simulink model "final_simulation"  (R2021b)
settings: Solver=ode8  StartTime=0.0  StopTime=T  FixedStep=0.1  RelTol=1e-3
values from neighbouring files (symbols this model uses):
  a_vec = 1./varVec    [variables.m]
  cutoff_omega = 0.1    [variables.m]
  date = date2jd([2021,2,23,0,0,0])    [variables.m]
  invJ = inv(J)    [variables.m]
  invJr = inv(Jr)    [variables.m]
  J = [Ixx 0 0; 0 Iyy 0; 0 0 Izz]    [variables.m]
  Jr = [Ir 0 0; 0 Ir 0; 0 0 Ir]    [variables.m]
  kd = 0    [variables.m]
  kdp = 0    [variables.m]
  ki = 0    [variables.m]
  kip = 1    [variables.m]
  komega = 0.01    [variables.m]
  kp = 20    [variables.m]
  kp1 = 0.2    [variables.m]
  kp2 = 2    [variables.m]
  kpp = 10    [variables.m]
  m_MT = 200    [variables.m]
  mu = astroConstants(13)    [variables.m]
  omega0 = [omegax0 omegay0 omegaz0]'    [variables.m]
  omegar0 = [omegaxr0 omegayr0 omegazr0]'    [variables.m]
  p = [0.05 0.05 0.05]'    [variables.m]
  q0 = [0 0 0 1]'    [variables.m]
  SstarsRef = [1/sqrt(3) 1 0; 1/sqrt(3) 0 1; 1/sqrt(3) 0 0]    [variables.m]
  theta0 = 2*atan(sqrt((1+en)/(1-en))*tan(E/2))    [variables.m]
undefined symbols (not defined in the file or in its folder): DiscIntNeverNeededParam, i, OM, om
libraries: matrix_library x7, my_math_ops x7, environment x5, simulink x4, vrlib x2, orbit x2, SENSORS x2, STATIC_ATT_DET x1, kinematic_transform x1
settings Model: Creator=paolo  LastModifiedBy=Davide

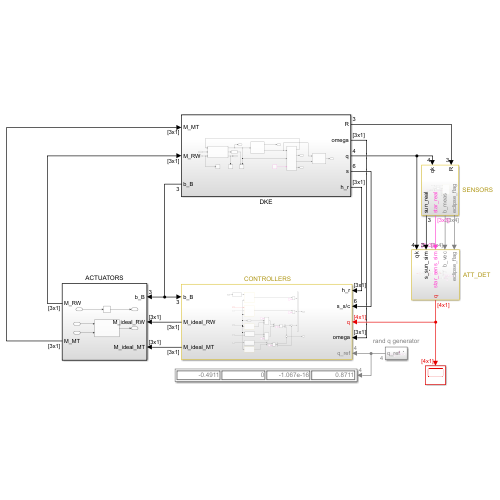
[thumbnail: Simulink's stored preview of the top-level diagram]
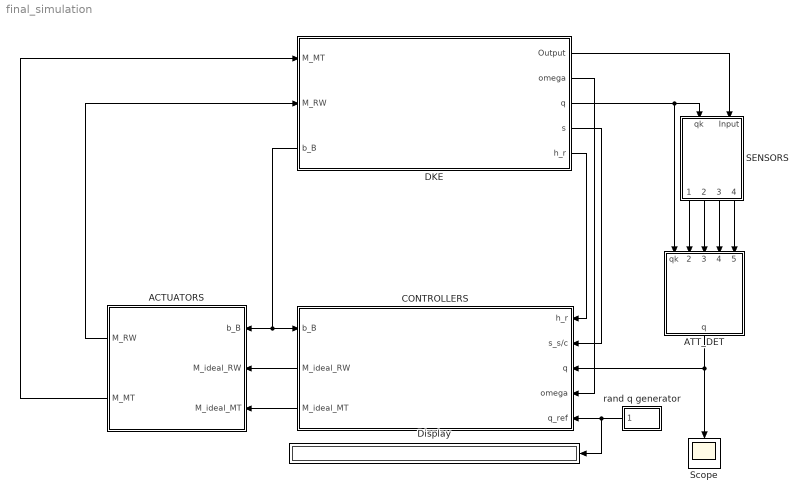
== system final_simulation ==
  " CONTROLLERS" : Subsystem
      settings: PortSchema="{\"entries\":[{\"content\":{\"sides\":[{\"content\":{\"connectorIds\":[\"In1\",\"In2\",\"In3\",\"In4\",\"In5\"]},\"type\":\"ConnectorPlacement.EquallySpacedRectSide\",\"uuid\":\"7eef0a68-69c2-4999-9870-ee920e7db8bb\"},{\"content\":{\"connectorIds\":[\"In6\",\"Out1\",\"Out2\"],\"side\":\"RIGHT\"},\"type\":\"ConnectorPlacement.EquallySpacedRectSide\",\"uuid\":\"b3de6d2c-2701-4d2f-a412-bdd263d79537\"},{\"content\":{\"connectorIds\":[],\"side\":\"TOP\"},\"type\":\"ConnectorPlacement.EquallySpacedRectSide\",\"uuid\":\"07183a01-e4e6-4ff7-8c71-3490d9a201db\"}]},\"type\":\"ConnectorPlacement.EquallySpacedConnector\",\"uuid\":\"cdaedd78-7c02-4158-8a0c-2b1dd6bc142b\"}],\"packageUris\":[\"http://schema.mathworks.com/mf0/Connector/R2020b\"],\"version\":\"1.0\"}"
  ACTUATORS : Subsystem
  ATT_DET : Subsystem
  DKE : Subsystem
      settings: PortSchema="{\"entries\":[{\"content\":{\"sides\":[{\"content\":{\"connectorIds\":[\"In1\",\"In2\",\"Out6\"]},\"type\":\"ConnectorPlacement.EquallySpacedRectSide\",\"uuid\":\"569b6a85-cacc-4d6a-9063-c3b1cb76f95a\"},{\"content\":{\"connectorIds\":[\"Out1\",\"Out2\",\"Out3\",\"Out4\",\"Out5\"],\"side\":\"RIGHT\"},\"type\":\"ConnectorPlacement.EquallySpacedRectSide\",\"uuid\":\"c98c0bd3-c24b-4331-a1c4-85d34b4b1026\"},{\"content\":{\"connectorIds\":[],\"side\":\"TOP\"},\"type\":\"ConnectorPlacement.EquallySpacedRectSide\",\"uuid\":\"0d550e56-de8b-41bd-9d95-3a45f35f27e4\"}]},\"type\":\"ConnectorPlacement.EquallySpacedConnector\",\"uuid\":\"b9a110d8-eb7f-46ee-8312-1f7318af1496\"}],\"packageUris\":[\"http://schema.mathworks.com/mf0/Connector/R2020b\"],\"version\":\"1.0\"}"
  Display : Display
  SENSORS : Subsystem
  Scope : Scope
  rand q generator : Subsystem
  wires:
  " CONTROLLERS"/2(M_ideal_MT) -> ACTUATORS/3(M_ideal_MT)
  DKE/2(omega) -> " CONTROLLERS"/4(omega)
  DKE/5(h_r) -> " CONTROLLERS"/1(h_r)
  DKE/3(q) -> ATT_DET/1(qk), SENSORS/1(qk)
  ACTUATORS/2(M_MT) -> DKE/1(M_MT)
  " CONTROLLERS"/1(M_ideal_RW) -> ACTUATORS/2(M_ideal_RW)
  DKE/6(b_B) -> ACTUATORS/1(b_B), " CONTROLLERS"/6(b_B)
  DKE/4(s) -> " CONTROLLERS"/2(s_s/c)
  ACTUATORS/1(M_RW) -> DKE/2(M_RW)
  ATT_DET/1(q) -> " CONTROLLERS"/3(q), Scope/1
  rand q generator/1(q_ref) -> " CONTROLLERS"/5(q_ref), Display/1
  SENSORS/1(sun_real) -> ATT_DET/2(s_sun_sim)
  SENSORS/2(star_real) -> ATT_DET/3(star_sens_sim)
  SENSORS/3(b_meas) -> ATT_DET/4(b_vec)
  DKE/1(Output) -> SENSORS/2(Input)
  SENSORS/4(Output) -> ATT_DET/5(Input)

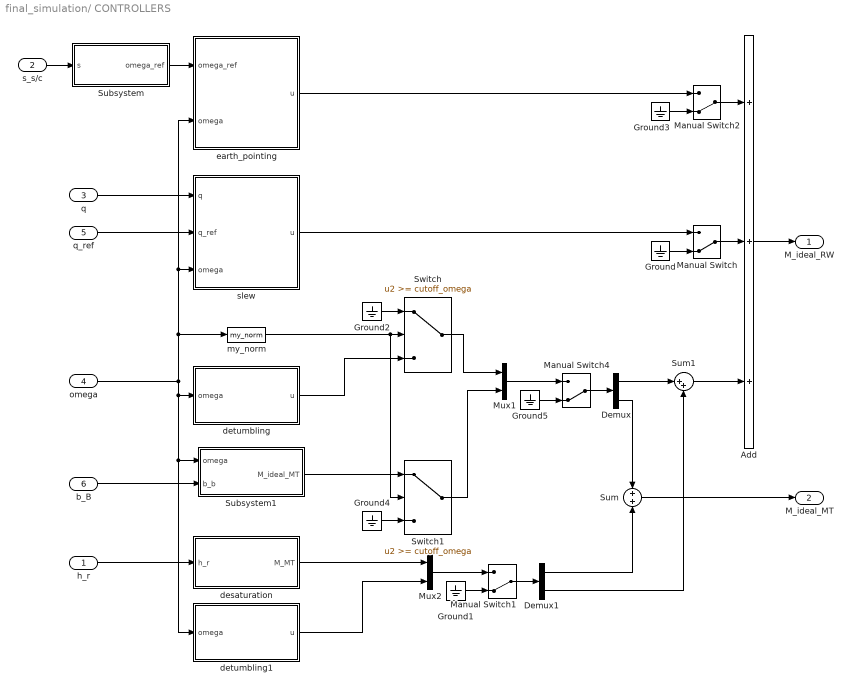
== system final_simulation/ CONTROLLERS ==
  h_r : Inport
  s_s/c : Inport  Port=2
  q : Inport  Port=3
  omega : Inport  Port=4
  q_ref : Inport  Port=5
  b_B : Inport  Port=6
  Add : Sum  Inputs=+++
  Demux : Demux  Outputs=2
  Demux1 : Demux  Outputs=2
  Ground{,1..5} (6 alike) : Ground
  Manual Switch{,1..2,4} (4 alike) : ManualSwitch  CurrentSetting=0
  Mux1 : Mux  Inputs=2
  Mux2 : Mux  Inputs=2
  Subsystem : Subsystem
  Subsystem1 : Subsystem
  Sum : Sum  Inputs=+|+
  Sum1 : Sum  Inputs=|++
  Switch : Switch  Threshold=cutoff_omega
  Switch1 : Switch  Threshold=cutoff_omega  ZeroCross=off
  desaturation : Subsystem
  detumbling : Subsystem
  detumbling1 : Subsystem
  earth_pointing : Subsystem
  my_norm : my_math_ops/my_norm  SystemSampleTime=-1  VariantActivationTime=update diagram  Latency=0  AutoFrameSizeCalculation=off
      settings: SourceProductName=My Mathematics Operations
  slew : Subsystem
  M_ideal_RW : Outport
  M_ideal_MT : Outport  Port=2
  wires:
  omega/1 -> detumbling/1(omega), detumbling1/1(omega), Subsystem1/1(omega), my_norm/1, earth_pointing/2(omega), slew/3(omega)
  Ground/1 -> Manual Switch/2
  Manual Switch/1 -> Add/2
  Add/1 -> M_ideal_RW/1
  q/1 -> slew/1(q)
  q_ref/1 -> slew/2(q_ref)
  slew/1(u) -> Manual Switch/1
  Ground3/1 -> Manual Switch2/2
  Manual Switch2/1 -> Add/1
  Subsystem/1(omega_ref) -> earth_pointing/1(omega_ref)
  earth_pointing/1(u) -> Manual Switch2/1
  s_s/c/1 -> Subsystem/1(s)
  Ground2/1 -> Switch/1
  my_norm/1 -> Switch1/2, Switch/2
  b_B/1 -> Subsystem1/2(b_b)
  Subsystem1/1(M_ideal_MT) -> Switch1/1
  Ground4/1 -> Switch1/3
  detumbling/1(u) -> Switch/3
  Switch/1 -> Mux1/1
  Switch1/1 -> Mux1/2
  Ground5/1 -> Manual Switch4/2
  Mux1/1 -> Manual Switch4/1
  Manual Switch4/1 -> Demux/1
  Demux/2 -> Sum/1
  Sum/1 -> M_ideal_MT/1
  h_r/1 -> desaturation/1(h_r)
  Mux2/1 -> Manual Switch1/1
  Manual Switch1/1 -> Demux1/1
  Ground1/1 -> Manual Switch1/2
  desaturation/1(M_MT) -> Mux2/1
  Demux1/1 -> Sum/2
  Demux/1 -> Sum1/1
  Sum1/1 -> Add/3
  detumbling1/1(u) -> Mux2/2
  Demux1/2 -> Sum1/2

== system final_simulation/ACTUATORS ==
  b_B : Inport
  M_ideal_RW : Inport  Port=2
  M_ideal_MT : Inport  Port=3
  Saturation : Saturate  UpperLimit=0.1  LowerLimit=-0.1
  Subsystem : Subsystem
  M_RW : Outport
  M_MT : Outport  Port=2
  wires:
  M_ideal_RW/1 -> Saturation/1
  Saturation/1 -> M_RW/1
  M_ideal_MT/1 -> Subsystem/1(M_ideal_MT)
  b_B/1 -> Subsystem/2(b_B)
  Subsystem/1(M_MT) -> M_MT/1

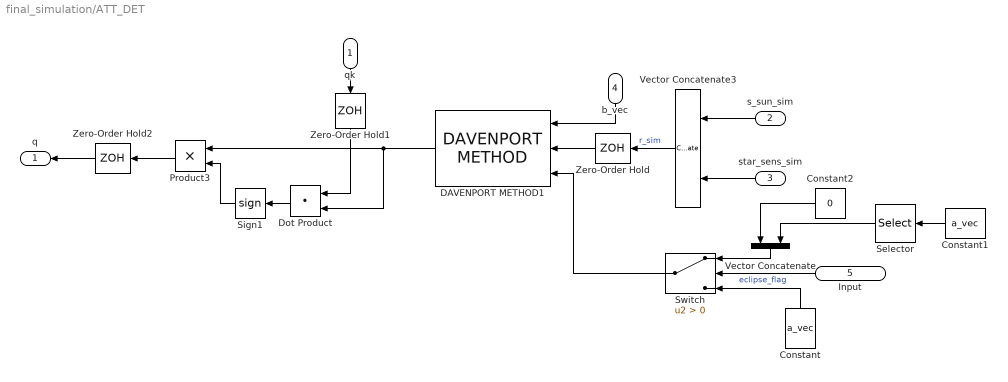
== system final_simulation/ATT_DET ==
  qk : Inport
  s_sun_sim : Inport  Port=2
  star_sens_sim : Inport  Port=3
  b_vec : Inport  Port=4
  Input : Inport  Port=5
  Constant : Constant  Value=a_vec
  Constant1 : Constant  Value=a_vec
  Constant2 : Constant  Value=0
  DAVENPORT METHOD1 : STATIC_ATT_DET/DAVENPORT METHOD  SystemSampleTime=-1  VariantActivationTime=update diagram  Latency=0  AutoFrameSizeCalculation=off
      settings: SourceProductName=Attitude Determination (static)
  Dot Product : DotProduct  InputSameDT=on  OutDataTypeStr=Inherit: Inherit via internal rule
  Product3 : Product
  Selector : Selector  InputPortWidth=4  IndexOptions=Index vector (dialog)  Indices=[2 3 4]  OutputSizes=1
  Sign1 : Signum
  Switch : Switch  Criteria=u2 > Threshold
  Vector Concatenate : Concatenate
  Vector Concatenate3 : Concatenate  Mode=Multidimensional array  ConcatenateDimension=2
  Zero-Order Hold : ZeroOrderHold  SampleTime=0.1
  Zero-Order Hold1 : ZeroOrderHold  SampleTime=0.1
  Zero-Order Hold2 : ZeroOrderHold  SampleTime=0.1
  q : Outport
  wires:
  star_sens_sim/1 -> Vector Concatenate3/2
  DAVENPORT METHOD1/1 -> Dot Product/2, Product3/1
  Sign1/1 -> Product3/2
  qk/1 -> Zero-Order Hold1/1
  Vector Concatenate3/1 -> Zero-Order Hold/1  "r_sim"
  Dot Product/1 -> Sign1/1
  s_sun_sim/1 -> Vector Concatenate3/1
  b_vec/1 -> DAVENPORT METHOD1/1
  Zero-Order Hold/1 -> DAVENPORT METHOD1/2
  Zero-Order Hold1/1 -> Dot Product/1
  Input/1 -> Switch/2  "eclipse_flag"
  Switch/1 -> DAVENPORT METHOD1/3
  Constant/1 -> Switch/3
  Constant1/1 -> Selector/1
  Selector/1 -> Vector Concatenate/2
  Constant2/1 -> Vector Concatenate/1
  Vector Concatenate/1 -> Switch/1
  Product3/1 -> Zero-Order Hold2/1
  Zero-Order Hold2/1 -> q/1

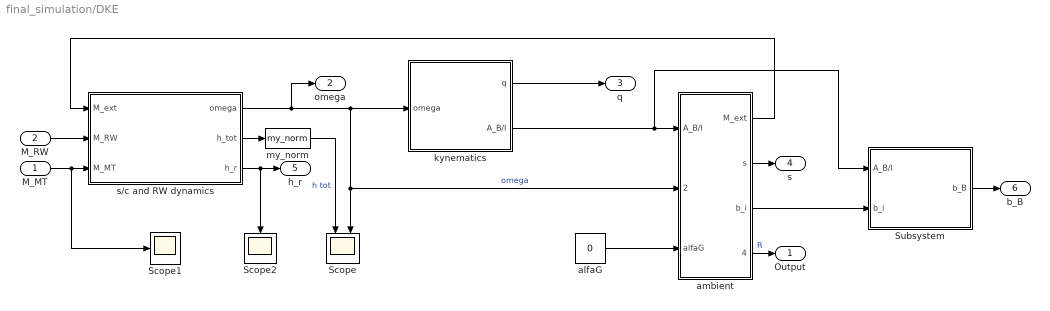
== system final_simulation/DKE ==
  M_MT : Inport
  M_RW : Inport  Port=2
  Scope : Scope  NumInputPorts=2
  Scope1 : Scope
  Scope2 : Scope
  Subsystem : Subsystem
  alfaG : Constant  Value=0
  ambient : Subsystem
  kynematics : Subsystem
  my_norm : my_math_ops/my_norm  SystemSampleTime=-1  VariantActivationTime=update diagram  Latency=0  AutoFrameSizeCalculation=off
      settings: SourceProductName=My Mathematics Operations
  s/c and RW dynamics : Subsystem
  Output : Outport
  omega : Outport  Port=2
  q : Outport  Port=3
  s : Outport  Port=4
  h_r : Outport  Port=5
  b_B : Outport  Port=6
  wires:
  s/c and RW dynamics/1(omega) -> Scope/2, ambient/2(omega), kynematics/1(omega), omega/1  "omega"
  kynematics/2(A_B/I) -> ambient/1(A_B/I), Subsystem/1(A_B/I)
  s/c and RW dynamics/2(h_tot) -> my_norm/1
  kynematics/1(q) -> q/1
  M_RW/1 -> s/c and RW dynamics/2(M_RW)
  ambient/1(M_ext) -> s/c and RW dynamics/1(M_ext)
  my_norm/1 -> Scope/1  "h tot"
  ambient/2(s) -> s/1
  alfaG/1 -> ambient/3(alfaG)
  ambient/3(b_i) -> Subsystem/2(b_i)
  M_MT/1 -> Scope1/1, s/c and RW dynamics/3(M_MT)
  Subsystem/1(b_B) -> b_B/1
  s/c and RW dynamics/3(h_r) -> Scope2/1, h_r/1
  ambient/4(Output) -> Output/1  "R"

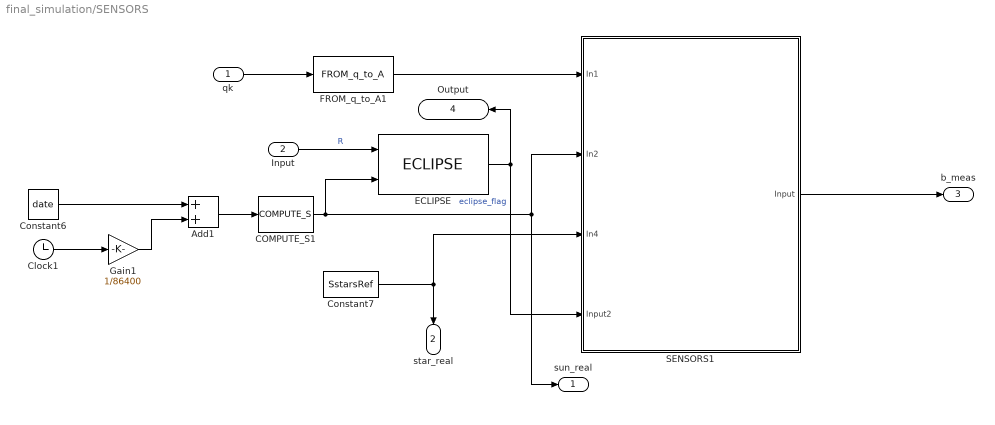
== system final_simulation/SENSORS ==
  qk : Inport
  Input : Inport  Port=2
  Add1 : Sum
  COMPUTE_S1 : environment/COMPUTE_S  SystemSampleTime=-1  VariantActivationTime=update diagram  Latency=0  AutoFrameSizeCalculation=off
      settings: SourceProductName=Environment
  Clock1 : Clock
  Constant6 : Constant  Value=date
  Constant7 : Constant  Value=SstarsRef
  ECLIPSE : environment/ECLIPSE  SystemSampleTime=-1  VariantActivationTime=update diagram  Latency=0  AutoFrameSizeCalculation=off
      settings: SourceProductName=Environment
  FROM_q_to_A1 : kinematic_transform/FROM_q_to_A  SystemSampleTime=-1  VariantActivationTime=update diagram  Latency=0  AutoFrameSizeCalculation=off
      settings: SourceProductName=Kinematic Transformation
  Gain1 : Gain  Gain=1/86400
  SENSORS1 : Subsystem
  sun_real : Outport
  star_real : Outport  Port=2
  b_meas : Outport  Port=3
  Output : Outport  Port=4
  wires:
  Gain1/1 -> Add1/2
  Constant7/1 -> star_real/1, SENSORS1/3(In4)
  Constant6/1 -> Add1/1
  FROM_q_to_A1/1 -> SENSORS1/1(In1)
  Add1/1 -> COMPUTE_S1/1
  Clock1/1 -> Gain1/1
  SENSORS1/1(Input) -> b_meas/1
  COMPUTE_S1/1 -> ECLIPSE/2, sun_real/1, SENSORS1/2(In2)
  qk/1 -> FROM_q_to_A1/1
  Input/1 -> ECLIPSE/1  "R"
  ECLIPSE/1 -> SENSORS1/4(Input2), Output/1  "eclipse_flag"

== system final_simulation/rand q generator ==
  Compare To Zero : simulink/Logic and Bit Operations/Compare To Zero  relop=>=  OutDataTypeStr=boolean
  Constant4 : Constant  Value=[rand(4,1)]
  Constant5 : Constant  Value=q0
  Constant8 : Constant  Value=randi([-1 1],4,1)
  Constant9 : Constant
  Gain2 : Gain  Gain=2
  Manual Switch : ManualSwitch
  Normalize Vector1 : vrlib/Utilities/Normalize Vector  maxzero=0
  Product2 : Product
  Subtract : Sum  Inputs=+-
  q_ref : Outport
  wires:
  Constant4/1 -> Normalize Vector1/1
  Normalize Vector1/1 -> Product2/1
  Constant8/1 -> Compare To Zero/1
  Constant9/1 -> Subtract/2
  Subtract/1 -> Product2/2
  Compare To Zero/1 -> Gain2/1
  Gain2/1 -> Subtract/1
  Manual Switch/1 -> q_ref/1
  Constant5/1 -> Manual Switch/2
  Product2/1 -> Manual Switch/1

== system final_simulation/ CONTROLLERS/Subsystem ==
  s : Inport
  Cross Product : matrix_library/Cross Product
      settings: SourceProductBaseCode=SL
  Demux : Demux  Outputs=2
  Divide : Product  Inputs=/*
  Ground : Ground
  Ground1 : Ground
  Mux : Mux  Inputs=3
  Scope : Scope
  Square : Math  Operator=square  SaturateOnIntegerOverflow=on
  my_norm : my_math_ops/my_norm  SystemSampleTime=-1  VariantActivationTime=update diagram  Latency=0  AutoFrameSizeCalculation=off
      settings: SourceProductName=My Mathematics Operations
  my_norm1 : my_math_ops/my_norm  SystemSampleTime=-1  VariantActivationTime=update diagram  Latency=0  AutoFrameSizeCalculation=off
      settings: SourceProductName=My Mathematics Operations
  omega_ref : Outport
  wires:
  s/1 -> Demux/1
  Demux/1 -> my_norm/1, Cross Product/1  "R"
  Demux/2 -> Cross Product/2  "V"
  Cross Product/1 -> my_norm1/1
  my_norm/1 -> Scope/1, Square/1
  Square/1 -> Divide/1
  my_norm1/1 -> Divide/2
  Mux/1 -> omega_ref/1
  Divide/1 -> Mux/3
  Ground/1 -> Mux/1
  Ground1/1 -> Mux/2

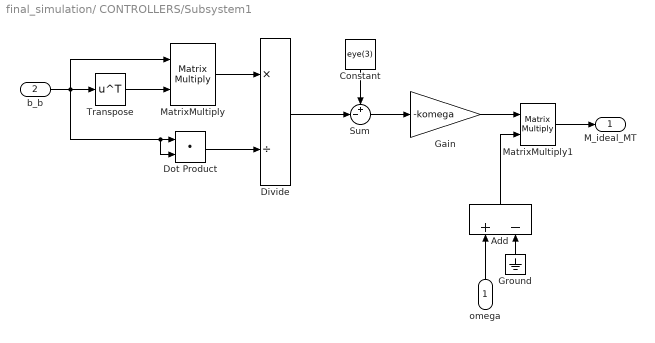
== system final_simulation/ CONTROLLERS/Subsystem1 ==
  omega : Inport
  b_b : Inport  Port=2
  Add : Sum  Inputs=+-
  Constant : Constant  Value=eye(3)
  Divide : Product  Inputs=*/
  Dot Product : DotProduct  InputSameDT=on  OutDataTypeStr=Inherit: Inherit via internal rule
  Gain : Gain  Gain=-komega
  Ground : Ground
  MatrixMultiply : Product  Multiplication=Matrix(*)
  MatrixMultiply1 : Product  Multiplication=Matrix(*)
  Sum : Sum  Inputs=+-|
  Transpose : Math  Operator=transpose  SaturateOnIntegerOverflow=on
  M_ideal_MT : Outport
  wires:
  Ground/1 -> Add/2
  omega/1 -> Add/1
  b_b/1 -> Dot Product/2, Dot Product/1, MatrixMultiply/1, Transpose/1
  Transpose/1 -> MatrixMultiply/2
  MatrixMultiply/1 -> Divide/1
  Dot Product/1 -> Divide/2
  Constant/1 -> Sum/1
  Divide/1 -> Sum/2
  Sum/1 -> Gain/1
  MatrixMultiply1/1 -> M_ideal_MT/1
  Gain/1 -> MatrixMultiply1/1
  Add/1 -> MatrixMultiply1/2

== system final_simulation/ CONTROLLERS/desaturation ==
  h_r : Inport
  Abs : Abs
  Constant : Constant
  Divide : Product  Inputs=*/
  Gain : Gain  Gain=-1/10
  MatrixMultiply : Product
  M_MT : Outport
  wires:
  Constant/1 -> Divide/1
  Divide/1 -> Abs/1
  Abs/1 -> MatrixMultiply/2
  MatrixMultiply/1 -> Gain/1
  h_r/1 -> MatrixMultiply/1, Divide/2
  Gain/1 -> M_MT/1

== system final_simulation/ CONTROLLERS/detumbling ==
  omega : Inport
  Add : Sum  Inputs=+-
  Discrete Derivative : simulink/Discrete/Discrete Derivative  gainval=1.0  ICPrevScaledInput=0.0  OutMin=[]  OutMax=[]  OutDataType=fixdt(1, 16)  OutScaling=2^-10  DoSatur=off
  Discrete-Time Integrator : DiscreteIntegrator  SampleTime=-1  ICPrevOutput=DiscIntNeverNeededParam  ICPrevScaledInput=DiscIntNeverNeededParam
  Gain : Gain  Gain=kp
  Gain1 : Gain  Gain=ki
  Gain2 : Gain  Gain=kd
  Ground : Ground
  Sum2 : Sum  Inputs=---
  u : Outport
  wires:
  Add/1 -> Gain/1, Discrete Derivative/1, Discrete-Time Integrator/1
  Ground/1 -> Add/2
  omega/1 -> Add/1
  Gain/1 -> Sum2/2
  Gain2/1 -> Sum2/3
  Gain1/1 -> Sum2/1
  Discrete-Time Integrator/1 -> Gain1/1
  Discrete Derivative/1 -> Gain2/1
  Sum2/1 -> u/1

== system final_simulation/ CONTROLLERS/detumbling1 ==
  omega : Inport
  Add : Sum  Inputs=+-
  Discrete Derivative : simulink/Discrete/Discrete Derivative  gainval=1.0  ICPrevScaledInput=0.0  OutMin=[]  OutMax=[]  OutDataType=fixdt(1, 16)  OutScaling=2^-10  DoSatur=off
  Discrete-Time Integrator : DiscreteIntegrator  SampleTime=-1  ICPrevOutput=DiscIntNeverNeededParam  ICPrevScaledInput=DiscIntNeverNeededParam
  Gain : Gain  Gain=kp
  Gain1 : Gain  Gain=ki
  Gain2 : Gain  Gain=kd
  Ground : Ground
  Sum2 : Sum  Inputs=---
  u : Outport
  wires:
  Add/1 -> Gain/1, Discrete Derivative/1, Discrete-Time Integrator/1
  Ground/1 -> Add/2
  omega/1 -> Add/1
  Gain/1 -> Sum2/2
  Gain2/1 -> Sum2/3
  Gain1/1 -> Sum2/1
  Discrete-Time Integrator/1 -> Gain1/1
  Discrete Derivative/1 -> Gain2/1
  Sum2/1 -> u/1

== system final_simulation/ CONTROLLERS/earth_pointing ==
  omega_ref : Inport
  omega : Inport  Port=2
  Add : Sum  Inputs=+-
  Discrete Derivative : simulink/Discrete/Discrete Derivative  gainval=1.0  ICPrevScaledInput=0.0  OutMin=[]  OutMax=[]  OutDataType=fixdt(1, 16)  OutScaling=2^-10  DoSatur=off
  Discrete-Time Integrator : DiscreteIntegrator  SampleTime=-1  ICPrevOutput=DiscIntNeverNeededParam  ICPrevScaledInput=DiscIntNeverNeededParam
  Gain : Gain  Gain=kpp
  Gain1 : Gain  Gain=kip
  Gain2 : Gain  Gain=kdp
  Sum2 : Sum  Inputs=---
  u : Outport
  wires:
  Add/1 -> Gain/1, Discrete Derivative/1, Discrete-Time Integrator/1
  Gain/1 -> Sum2/2
  Sum2/1 -> u/1
  omega/1 -> Add/1
  Discrete-Time Integrator/1 -> Gain1/1
  Gain1/1 -> Sum2/1
  omega_ref/1 -> Add/2
  Gain2/1 -> Sum2/3
  Discrete Derivative/1 -> Gain2/1

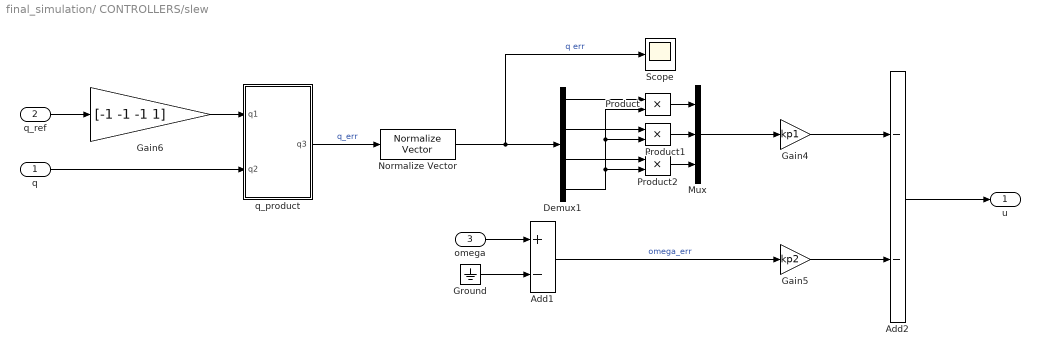
== system final_simulation/ CONTROLLERS/slew ==
  q : Inport
  q_ref : Inport  Port=2
  omega : Inport  Port=3
  Add1 : Sum  Inputs=+-
  Add2 : Sum  Inputs=--
  Demux1 : Demux
  Gain4 : Gain  Gain=kp1
  Gain5 : Gain  Gain=kp2
  Gain6 : Gain  Gain=[-1 -1 -1 1]
  Ground : Ground
  Mux : Mux  Inputs=3
  Normalize Vector : vrlib/Utilities/Normalize Vector  maxzero=0
  Product : Product
  Product1 : Product
  Product2 : Product
  Scope : Scope
  q_product : Subsystem
  u : Outport
  wires:
  omega/1 -> Add1/1
  Ground/1 -> Add1/2
  Add1/1 -> Gain5/1  "omega_err"
  Gain5/1 -> Add2/2
  Add2/1 -> u/1
  Gain4/1 -> Add2/1
  Normalize Vector/1 -> Scope/1, Demux1/1  "q err"
  Demux1/4 -> Product/2, Product1/2, Product2/2
  Mux/1 -> Gain4/1
  q_ref/1 -> Gain6/1
  Gain6/1 -> q_product/1(q1)
  q/1 -> q_product/2(q2)
  q_product/1(q3) -> Normalize Vector/1  "q_err"
  Product/1 -> Mux/1
  Product1/1 -> Mux/2
  Product2/1 -> Mux/3
  Demux1/3 -> Product2/1
  Demux1/2 -> Product1/1
  Demux1/1 -> Product/1

== system final_simulation/ACTUATORS/Subsystem ==
  M_ideal_MT : Inport
  b_B : Inport  Port=2
  Cross Product : matrix_library/Cross Product
      settings: SourceProductBaseCode=SL
  Cross Product1 : matrix_library/Cross Product
      settings: SourceProductBaseCode=SL
  Divide : Product  Inputs=*/
  Dot Product : DotProduct  InputSameDT=on  OutDataTypeStr=Inherit: Inherit via internal rule
  Saturation : Saturate  UpperLimit=m_MT  LowerLimit=-m_MT
  Scope : Scope
  Scope1 : Scope  NumInputPorts=2
  M_MT : Outport
  wires:
  b_B/1 -> Cross Product/1, Cross Product1/2, Dot Product/2, Dot Product/1  "b_B"
  M_ideal_MT/1 -> Scope1/2, Cross Product/2
  Cross Product/1 -> Divide/1
  Dot Product/1 -> Divide/2
  Cross Product1/1 -> Scope1/1, M_MT/1
  Divide/1 -> Saturation/1
  Saturation/1 -> Scope/1, Cross Product1/1  "d_B"

== system final_simulation/DKE/Subsystem ==
  A_B/I : Inport
  b_i : Inport  Port=2
  MatrixMultiply : Product  Multiplication=Matrix(*)
  b_B : Outport
  wires:
  A_B/I/1 -> MatrixMultiply/1
  b_i/1 -> MatrixMultiply/2
  MatrixMultiply/1 -> b_B/1  "b_B"

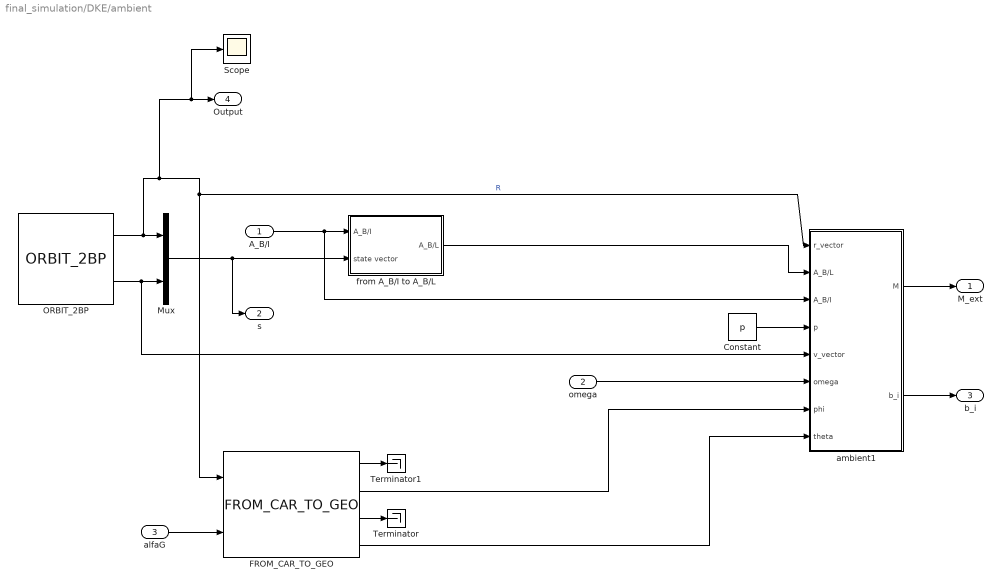
== system final_simulation/DKE/ambient ==
  A_B/I : Inport
  omega : Inport  Port=2
  alfaG : Inport  Port=3
  Constant : Constant  Value=p
  FROM_CAR_TO_GEO : orbit/FROM_CAR_TO_GEO  SystemSampleTime=-1  VariantActivationTime=update diagram  Latency=0  AutoFrameSizeCalculation=off
      settings: SourceProductName=Orbit
  Mux : Mux  Inputs=2
  ORBIT_2BP : orbit/ORBIT_2BP  SystemSampleTime=-1  VariantActivationTime=update diagram  Latency=0  AutoFrameSizeCalculation=off
      settings: SourceProductName=Orbit
  Scope : Scope
  Terminator : Terminator
  Terminator1 : Terminator
  ambient1 : Subsystem
  from A_B/I to A_B/L : Subsystem
  M_ext : Outport
  s : Outport  Port=2
  b_i : Outport  Port=3
  Output : Outport  Port=4
  wires:
  ORBIT_2BP/1 -> Scope/1, Output/1, ambient1/1(r_vector), FROM_CAR_TO_GEO/1, Mux/1  "R"
  ORBIT_2BP/2 -> ambient1/5(v_vector), Mux/2
  Mux/1 -> s/1, from A_B/I to A_B/L/2(state vector)
  A_B/I/1 -> ambient1/3(A_B/I), from A_B/I to A_B/L/1(A_B/I)
  alfaG/1 -> FROM_CAR_TO_GEO/2
  FROM_CAR_TO_GEO/3 -> Terminator/1
  FROM_CAR_TO_GEO/1 -> Terminator1/1
  ambient1/1(M) -> M_ext/1
  from A_B/I to A_B/L/1(A_B/L) -> ambient1/2(A_B/L)
  FROM_CAR_TO_GEO/2 -> ambient1/7(phi)
  FROM_CAR_TO_GEO/4 -> ambient1/8(theta)
  omega/1 -> ambient1/6(omega)
  Constant/1 -> ambient1/4(p)
  ambient1/2(b_i) -> b_i/1

== system final_simulation/DKE/kynematics ==
  omega : Inport
  kynematics q : Subsystem
  q to A_B/I : Subsystem
  q : Outport
  A_B/I : Outport  Port=2
  wires:
  omega/1 -> kynematics q/1(omega)
  kynematics q/1(q) -> q to A_B/I/1(q), q/1
  q to A_B/I/1(Aq) -> A_B/I/1

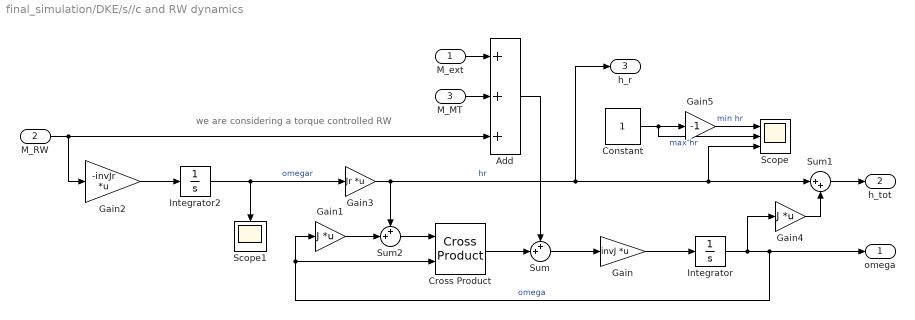
== system final_simulation/DKE/s//c and RW dynamics ==
  note: we are considering a torque controlled RW
  M_ext : Inport
  M_RW : Inport  Port=2
  M_MT : Inport  Port=3
  Add : Sum  Inputs=+++
  Constant : Constant
  Cross Product : matrix_library/Cross Product
      settings: SourceProductBaseCode=SL
  Gain : Gain  Gain=invJ  Multiplication=Matrix(K*u)
  Gain1 : Gain  Gain=J  Multiplication=Matrix(K*u)
  Gain2 : Gain  Gain=-invJr  Multiplication=Matrix(K*u)
  Gain3 : Gain  Gain=Jr  Multiplication=Matrix(K*u)
  Gain4 : Gain  Gain=J  Multiplication=Matrix(K*u)
  Gain5 : Gain  Gain=-1
  Integrator : Integrator  InitialCondition=omega0
  Integrator2 : Integrator  InitialCondition=omegar0
  Scope : Scope  NumInputPorts=3
  Scope1 : Scope
  Sum : Sum  Inputs=++|
  Sum1 : Sum  Inputs=|++
  Sum2 : Sum  Inputs=++|
  omega : Outport
  h_tot : Outport  Port=2
  h_r : Outport  Port=3
  wires:
  Integrator/1 -> omega/1, Gain1/1, Cross Product/2, Gain4/1  "omega"
  Cross Product/1 -> Sum/2
  Sum/1 -> Gain/1
  Gain/1 -> Integrator/1
  Sum2/1 -> Cross Product/1
  Gain1/1 -> Sum2/2
  M_RW/1 -> Add/3, Gain2/1
  Gain2/1 -> Integrator2/1
  Gain3/1 -> Sum2/1, Scope/3, Sum1/1, h_r/1  "hr"
  Integrator2/1 -> Gain3/1, Scope1/1  "omegar"
  Gain4/1 -> Sum1/2
  Sum1/1 -> h_tot/1
  Add/1 -> Sum/1
  Constant/1 -> Gain5/1, Scope/2  "max hr"
  M_ext/1 -> Add/1
  Gain5/1 -> Scope/1  "min hr"
  M_MT/1 -> Add/2

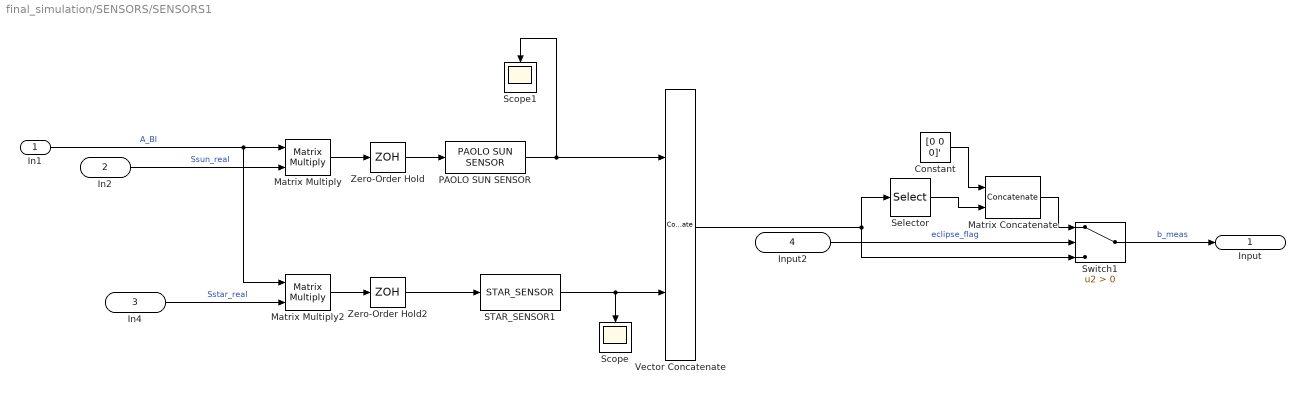
== system final_simulation/SENSORS/SENSORS1 ==
  In1 : Inport
  In2 : Inport  Port=2
  In4 : Inport  Port=3
  Input2 : Inport  Port=4
  Constant : Constant  Value=[0 0 0]'
  Matrix Concatenate : Concatenate  Mode=Multidimensional array  ConcatenateDimension=2
  Matrix Multiply : Product  Multiplication=Matrix(*)
  Matrix Multiply2 : Product  Multiplication=Matrix(*)
  PAOLO SUN SENSOR : SENSORS/PAOLO SUN SENSOR  SystemSampleTime=-1  VariantActivationTime=update diagram  Latency=0  AutoFrameSizeCalculation=off
      settings: SourceProductName=Sensors
  STAR_SENSOR1 : SENSORS/STAR_SENSOR  SystemSampleTime=-1  VariantActivationTime=update diagram  Latency=0  AutoFrameSizeCalculation=off
      settings: SourceProductName=Sensors
  Scope : Scope
  Scope1 : Scope
  Selector : Selector  NumberOfDimensions=2  InputPortWidth=3  IndexOptions=Index vector (dialog),Index vector (dialog)  Indices=[1 2 3],[2 3 4]  OutputSizes=1,1
  Switch1 : Switch  Criteria=u2 > Threshold
  Vector Concatenate : Concatenate  Mode=Multidimensional array  ConcatenateDimension=2
  Zero-Order Hold : ZeroOrderHold  SampleTime=0.1
  Zero-Order Hold2 : ZeroOrderHold  SampleTime=0.2
  Input : Outport
  wires:
  Zero-Order Hold2/1 -> STAR_SENSOR1/1
  STAR_SENSOR1/1 -> Vector Concatenate/2, Scope/1
  In1/1 -> Matrix Multiply2/1, Matrix Multiply/1  "A_BI"
  In4/1 -> Matrix Multiply2/2  "Sstar_real"
  Matrix Multiply2/1 -> Zero-Order Hold2/1
  In2/1 -> Matrix Multiply/2  "Ssun_real"
  Matrix Multiply/1 -> Zero-Order Hold/1
  Vector Concatenate/1 -> Switch1/3, Selector/1
  Zero-Order Hold/1 -> PAOLO SUN SENSOR/1
  PAOLO SUN SENSOR/1 -> Vector Concatenate/1, Scope1/1
  Input2/1 -> Switch1/2  "eclipse_flag"
  Switch1/1 -> Input/1  "b_meas"
  Selector/1 -> Matrix Concatenate/2
  Constant/1 -> Matrix Concatenate/1
  Matrix Concatenate/1 -> Switch1/1

== system final_simulation/ CONTROLLERS/slew/q_product ==
  q1 : Inport
  q2 : Inport  Port=2
  Add : Sum  Inputs=3
  Add1 : Sum  Inputs=+-
  Cross Product : matrix_library/Cross Product
      settings: SourceProductBaseCode=SL
  Dot Product : DotProduct  InputSameDT=on  OutDataTypeStr=Inherit: Inherit via internal rule
  Product : Product
  Product1 : Product
  Product2 : Product
  Subsystem : Subsystem
  Subsystem1 : Subsystem
  Vector Concatenate : Concatenate
  q3 : Outport
  wires:
  Product/1 -> Add/2
  Subsystem1/2(n_ref) -> Product1/1, Product2/2
  Subsystem/1(g) -> Dot Product/1, Product1/2, Cross Product/1
  Cross Product/1 -> Add/1
  q1/1 -> Subsystem/1(q)
  Subsystem1/1(g_ref) -> Dot Product/2, Product/2, Cross Product/2
  Add/1 -> Vector Concatenate/1
  Product1/1 -> Add/3
  Dot Product/1 -> Add1/2
  Subsystem/2(n) -> Product2/1, Product/1
  Product2/1 -> Add1/1
  Add1/1 -> Vector Concatenate/2
  q2/1 -> Subsystem1/1(q_ref)
  Vector Concatenate/1 -> q3/1

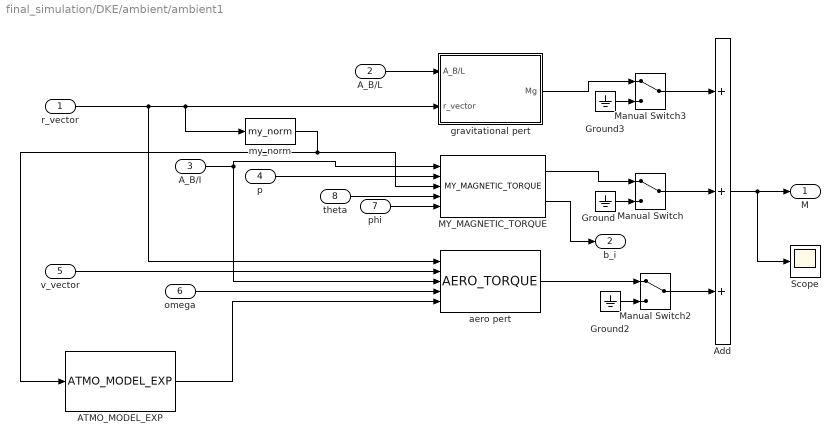
== system final_simulation/DKE/ambient/ambient1 ==
  r_vector : Inport
  A_B/L : Inport  Port=2
  A_B/I : Inport  Port=3
  p : Inport  Port=4
  v_vector : Inport  Port=5
  omega : Inport  Port=6
  phi : Inport  Port=7
  theta : Inport  Port=8
  ATMO_MODEL_EXP : environment/ATMO_MODEL_EXP  SystemSampleTime=-1  VariantActivationTime=update diagram  Latency=0  AutoFrameSizeCalculation=off
      settings: SourceProductName=Environment
  Add : Sum  Inputs=+++
  Ground : Ground
  Ground2 : Ground
  Ground3 : Ground
  MY_MAGNETIC_TORQUE : environment/MY_MAGNETIC_TORQUE  SystemSampleTime=-1  VariantActivationTime=update diagram  Latency=0  AutoFrameSizeCalculation=off
      settings: SourceProductName=Environment
  Manual Switch : ManualSwitch
  Manual Switch2 : ManualSwitch
  Manual Switch3 : ManualSwitch
  Scope : Scope
  aero pert : environment/AERO_TORQUE  SystemSampleTime=-1  VariantActivationTime=update diagram  Latency=0  AutoFrameSizeCalculation=off
      settings: SourceProductName=Environment
  gravitational pert : Subsystem
  my_norm : my_math_ops/my_norm  SystemSampleTime=-1  VariantActivationTime=update diagram  Latency=0  AutoFrameSizeCalculation=off
      settings: SourceProductName=My Mathematics Operations
  M : Outport
  b_i : Outport  Port=2
  wires:
  p/1 -> MY_MAGNETIC_TORQUE/2
  theta/1 -> MY_MAGNETIC_TORQUE/4
  ATMO_MODEL_EXP/1 -> aero pert/5
  MY_MAGNETIC_TORQUE/1 -> Manual Switch/1
  omega/1 -> aero pert/4
  phi/1 -> MY_MAGNETIC_TORQUE/5
  aero pert/1 -> Manual Switch2/1
  gravitational pert/1(Mg) -> Manual Switch3/1
  A_B/I/1 -> MY_MAGNETIC_TORQUE/1, aero pert/3
  Ground2/1 -> Manual Switch2/2
  Manual Switch/1 -> Add/2
  v_vector/1 -> aero pert/2
  Ground3/1 -> Manual Switch3/2
  Add/1 -> Scope/1, M/1
  my_norm/1 -> MY_MAGNETIC_TORQUE/3, ATMO_MODEL_EXP/1
  r_vector/1 -> aero pert/1, my_norm/1, gravitational pert/2(r_vector)
  Ground/1 -> Manual Switch/2
  Manual Switch2/1 -> Add/3
  A_B/L/1 -> gravitational pert/1(A_B/L)
  Manual Switch3/1 -> Add/1
  MY_MAGNETIC_TORQUE/2 -> b_i/1

== system final_simulation/DKE/ambient/from A_B//I to A_B//L ==
  A_B/I : Inport
  state vector : Inport  Port=2
  A_I_LVLH1 : Subsystem
  Demux : Demux  Outputs=2
  MatrixMultiply : Product  Multiplication=Matrix(*)
  Subsystem : Subsystem
  Terminator : Terminator
  A_B/L : Outport
  wires:
  MatrixMultiply/1 -> A_B/L/1
  A_B/I/1 -> MatrixMultiply/1
  A_I_LVLH1/1(Out1) -> MatrixMultiply/2  "A_I/L"
  Subsystem/2(Out2) -> Terminator/1  "omega_L"
  Subsystem/1(Out1) -> A_I_LVLH1/1(Input)
  Demux/1 -> Subsystem/1(a)
  Demux/2 -> Subsystem/2(b)
  state vector/1 -> Demux/1

== system final_simulation/DKE/kynematics/kynematics q ==
  omega : Inport
  Add : Sum  Inputs=+++
  Demux : Demux  Outputs=3
  Gain : Gain  Gain=[0 0 0 1; 0 0 1 0; 0 -1 0 0; -1 0 0 0]
  Gain1 : Gain  Gain=[0 0 -1 0; 0 0 0 1; 1 0 0 0; 0 -1 0 0]
  Gain2 : Gain  Gain=[0 1 0 0; -1 0 0 0; 0 0 0 1; 0 0 -1 0]
  Gain3 : Gain  Gain=1/2
  Integrator : Integrator  InitialCondition=q0
  Product : Product  Multiplication=Matrix(*)
  normalization : Subsystem
  q : Outport
  wires:
  Product/1 -> Integrator/1  "dq"
  Gain/1 -> Add/1
  Gain3/1 -> Product/1
  Add/1 -> Gain3/1
  Gain2/1 -> Add/3
  Gain1/1 -> Add/2
  Demux/3 -> Gain2/1
  Demux/1 -> Gain/1
  Demux/2 -> Gain1/1
  omega/1 -> Demux/1
  Integrator/1 -> normalization/1(q0)
  normalization/1(q) -> Product/2, q/1

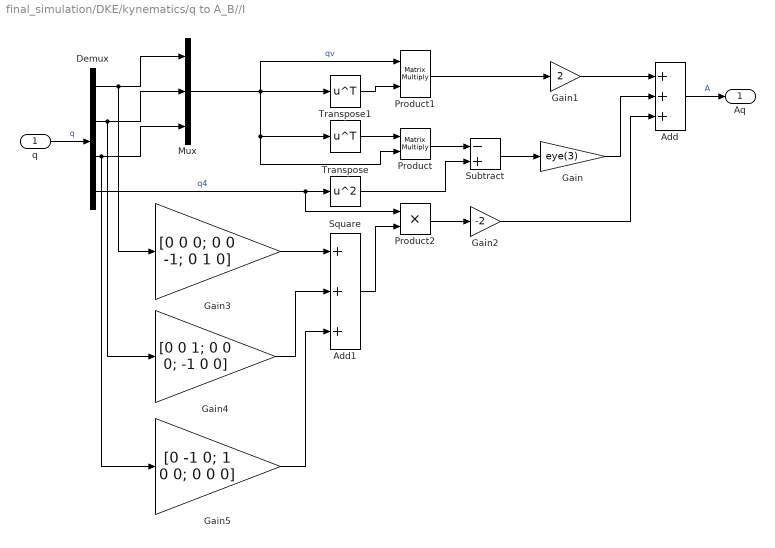
== system final_simulation/DKE/kynematics/q to A_B//I ==
  q : Inport
  Add : Sum  Inputs=+++
  Add1 : Sum  Inputs=+++
  Demux : Demux
  Gain : Gain  Gain=eye(3)
  Gain1 : Gain  Gain=2
  Gain2 : Gain  Gain=-2
  Gain3 : Gain  Gain=[0 0 0; 0 0 -1; 0 1 0]
  Gain4 : Gain  Gain=[0 0 1; 0 0 0; -1 0 0]
  Gain5 : Gain  Gain=[0 -1 0; 1 0 0; 0 0 0]
  Mux : Mux  Inputs=3
  Product : Product  Multiplication=Matrix(*)
  Product1 : Product  Multiplication=Matrix(*)
  Product2 : Product
  Square : Math  Operator=square  SaturateOnIntegerOverflow=on
  Subtract : Sum  Inputs=-+
  Transpose : Math  Operator=transpose  SaturateOnIntegerOverflow=on
  Transpose1 : Math  Operator=transpose  SaturateOnIntegerOverflow=on
  Aq : Outport
  wires:
  Product/1 -> Subtract/1
  Gain4/1 -> Add1/2
  Add/1 -> Aq/1  "A"
  Transpose/1 -> Product/1
  Square/1 -> Subtract/2
  Product1/1 -> Gain1/1
  Gain/1 -> Add/2
  Gain3/1 -> Add1/1
  Product2/1 -> Gain2/1
  Gain2/1 -> Add/3
  Gain1/1 -> Add/1
  Gain5/1 -> Add1/3
  q/1 -> Demux/1  "q"
  Add1/1 -> Product2/2
  Mux/1 -> Product/2, Transpose/1, Transpose1/1, Product1/1  "qv"
  Subtract/1 -> Gain/1
  Demux/4 -> Product2/1, Square/1  "q4"
  Demux/3 -> Gain5/1, Mux/3
  Transpose1/1 -> Product1/2
  Demux/2 -> Gain4/1, Mux/2
  Demux/1 -> Gain3/1, Mux/1

== system final_simulation/ CONTROLLERS/slew/q_product/Subsystem ==
  q : Inport
  Demux : Demux
  Mux : Mux  Inputs=3
  g : Outport
  n : Outport  Port=2
  wires:
  Demux/2 -> Mux/2
  q/1 -> Demux/1
  Demux/3 -> Mux/3
  Demux/1 -> Mux/1
  Mux/1 -> g/1
  Demux/4 -> n/1

== system final_simulation/ CONTROLLERS/slew/q_product/Subsystem1 ==
  q_ref : Inport
  Demux : Demux
  Mux : Mux  Inputs=3
  g_ref : Outport
  n_ref : Outport  Port=2
  wires:
  Demux/2 -> Mux/2
  q_ref/1 -> Demux/1
  Demux/3 -> Mux/3
  Demux/1 -> Mux/1
  Mux/1 -> g_ref/1
  Demux/4 -> n_ref/1

== system final_simulation/DKE/ambient/ambient1/gravitational pert ==
  A_B/L : Inport
  r_vector : Inport  Port=2
  Constant : Constant  Value=[1 0 0]
  Constant1 : Constant  Value=3
  Cross Product1 : matrix_library/Cross Product
      settings: SourceProductBaseCode=SL
  Divide : Product  Inputs=/*
  Dot Product : DotProduct  InputSameDT=on  OutDataTypeStr=Inherit: Inherit via internal rule
  Gain3 : Gain  Gain=J  Multiplication=Matrix(K*u)
  Gain4 : Gain  Gain=-3*mu
  Power : Math  Operator=pow  SaturateOnIntegerOverflow=on
  Product : Product  Multiplication=Matrix(*)
  Square Root : Sqrt  SaturateOnIntegerOverflow=on
  Mg : Outport
  wires:
  Cross Product1/1 -> Gain4/1
  Product/1 -> Cross Product1/2, Gain3/1
  A_B/L/1 -> Product/1
  Constant/1 -> Product/2
  Gain3/1 -> Cross Product1/1
  Square Root/1 -> Power/1
  Gain4/1 -> Divide/2
  Constant1/1 -> Power/2
  Power/1 -> Divide/1
  Divide/1 -> Mg/1
  r_vector/1 -> Dot Product/2, Dot Product/1
  Dot Product/1 -> Square Root/1

== system final_simulation/DKE/ambient/from A_B//I to A_B//L/A_I_LVLH1 ==
  note: i need the orbital paramaters
  note: i need the orbital paramaters
  Input : Inport
  Product : Product  Multiplication=Matrix(*)
  Product1 : Product  Multiplication=Matrix(*)
  R1 : Constant  Value="[cos(OM)  sin(OM) 0; -sin(OM) cos(OM) 0; 0 0 1]"
  R2 : Constant  Value=[1 0 0; 0 cos(i) sin(i); 0 -sin(i) cos(i)]
  R3 : Subsystem
  Transpose : Math  Operator=transpose  SaturateOnIntegerOverflow=on
  Out1 : Outport
  wires:
  Transpose/1 -> Out1/1
  Product/1 -> Product1/1
  R2/1 -> Product/2
  Input/1 -> R3/1(w_I_norm)  "w_I_norm"
  Product1/1 -> Transpose/1
  R1/1 -> Product1/2
  R3/1(Output) -> Product/1

== system final_simulation/DKE/ambient/from A_B//I to A_B//L/Subsystem ==
  note: for the general case in which h not constant (J2 perturbed orbit)
  a : Inport
  b : Inport  Port=2
  Constant : Constant  Value=[0 0 1]'
  Cross Product : matrix_library/Cross Product
      settings: SourceProductBaseCode=SL
  Divide2 : Product  Inputs=/*
  Product7 : Product
  Square1 : Math  Operator=square  SaturateOnIntegerOverflow=on
  my_norm : my_math_ops/my_norm  SystemSampleTime=-1  VariantActivationTime=update diagram  Latency=0  AutoFrameSizeCalculation=off
      settings: SourceProductName=My Mathematics Operations
  my_norm4 : my_math_ops/my_norm  SystemSampleTime=-1  VariantActivationTime=update diagram  Latency=0  AutoFrameSizeCalculation=off
      settings: SourceProductName=My Mathematics Operations
  Out1 : Outport
  Out2 : Outport  Port=2
  wires:
  my_norm/1 -> Square1/1  "Rnorm"
  Constant/1 -> Product7/2
  Square1/1 -> Divide2/1
  b/1 -> Cross Product/2  "V"
  Divide2/1 -> Out1/1, Product7/1  "w_l_norm"
  my_norm4/1 -> Divide2/2  "h_norm_orb"
  a/1 -> my_norm/1, Cross Product/1  "R"
  Cross Product/1 -> my_norm4/1  "h_orb"
  Product7/1 -> Out2/1  "w_L"

== system final_simulation/DKE/kynematics/kynematics q/normalization ==
  q0 : Inport
  Divide : Product  Inputs=*/
  Dot Product : DotProduct  InputSameDT=on  OutDataTypeStr=Inherit: Inherit via internal rule
  Sqrt : Sqrt  SaturateOnIntegerOverflow=on
  q : Outport
  wires:
  Dot Product/1 -> Sqrt/1
  q0/1 -> Dot Product/1, Dot Product/2, Divide/1
  Sqrt/1 -> Divide/2
  Divide/1 -> q/1

== system final_simulation/DKE/ambient/from A_B//I to A_B//L/A_I_LVLH1/R3 ==
  w_I_norm : Inport
  Add : Sum
  Add1 : Sum  Inputs=+++
  Clock : Clock
  Constant2 : Constant  Value=[0 0 0; 0 0 0; 0 0 1]
  Constant3 : Constant  Value=om + theta0
  Cos : Trigonometry  Operator=cos
  Gain : Gain  Gain=[1 0 0; 0 1 0; 0 0 0]
  Gain1 : Gain  Gain=[0 1 0; -1 0 0; 0 0 0]
  Product1 : Product
  Sin : Trigonometry
  Output : Outport
  wires:
  Clock/1 -> Product1/1
  Product1/1 -> Add/1
  Gain/1 -> Add1/1
  Add1/1 -> Output/1  "R3"
  Add/1 -> Sin/1, Cos/1
  Gain1/1 -> Add1/2
  Cos/1 -> Gain/1
  Constant3/1 -> Add/2
  Sin/1 -> Gain1/1
  w_I_norm/1 -> Product1/2
  Constant2/1 -> Add1/3
